simulink model "Ecuacion_Diferencial_Ejercicio_3"  (R2017b)
settings: Solver=ode1  StartTime=0.0  StopTime=10.0  FixedStep=0.001  RelTol=1e-3
settings Model: Creator=Elmer  LastModifiedBy=Elmer

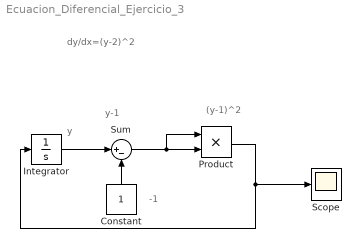
== system Ecuacion_Diferencial_Ejercicio_3 ==
  note: y-1
  note: dy/dx=(y-2)^2
  note: -1
  note: y
  note: (y-1)^2
  Constant : Constant
  Integrator : Integrator  InitialCondition=0.5
  Product : Product
  Scope : Scope
  Sum : Sum  Inputs=|+-
  wires:
  Constant/1 -> Sum/2
  Integrator/1 -> Sum/1
  Product/1 -> Scope/1, Integrator/1
  Sum/1 -> Product/2, Product/1
